simulink model "heli"  (R2020a)
settings: Solver=FixedStepAuto  StartTime=0  StopTime=Ts  FixedStep=0.0025  MaxStep=0.01  RelTol=1e-3  AbsTol=1e-3
values from neighbouring files (symbols this model uses):
  A_Fxyz_uvw_pqr = A([1 2 3],[1 2 3 4 5 6])    [heli_init.m]
  A_Mxyz_uvw_pqr = A([4 5 6],[1 2 3 4 5 6])    [heli_init.m]
  B_Fxyz_u_cont = B([1 2 3],[1 2 3 4])    [heli_init.m]
  B_Mxyz_u_cont = B([4 5 6],[1 2 3 4])    [heli_init.m]
  DCM_0 = [1 0 0 ... (first row only)    [heli_init.m]
  Dir_w = 0*[1 1 1 1 1 1]    [heli_init.m]
  East_0 = 0    [heli_init.m]
  h_0 = 0    [heli_init.m]
  hw = [0 200 5000 10000 15000 20000]    [heli_init.m]
  hw_gust = [0 1 h_island h_island+1 5000]    [heli_init.m]
  ic_euler_ang = zeros(3,1)    [heli_init.m]
  ic_U = sqrt(ic_u^2+ic_v^2+ic_w^2)    [heli_init.m]
  ic_v = 0.0000    (= 0)    [heli_init.m]
  ic_w = 0.0000    (= 0)    [heli_init.m]
  K_gust = 0    [heli_init.m]
  K_gust_factor = [1.1 1 .5 0.25 0]    [heli_init.m]
  M = 1    [heli_init.m]
  North_0 = 0    [heli_init.m]
  Pit_ic = 0    [heli_init.m]
  Psi = 353*pi/180.0    (= 6.16101225954)    [heli_init.m]
  Roll_ic = 0    [heli_init.m]
  Th_wind_limit = 40    [heli_init.m]
  Vw = 15*[1 1 1 1 1 1]    [heli_init.m]
  W_GUST = .8    (= 0.8)    [heli_init.m]
libraries: aerolibobsolete x2, AP_Conector x2, aerolibasang x1, aerolibwind2 x1

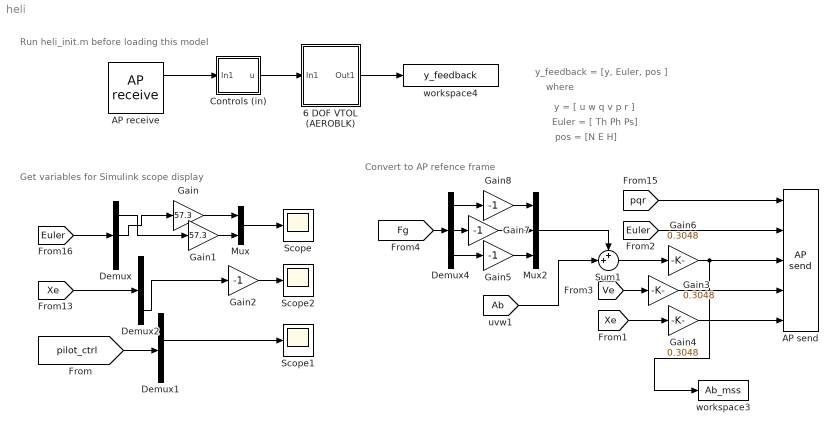
== system heli ==
  note: Run heli_init.m before loading this model
  note: Convert to AP refence frame
  note: Get variables for Simulink scope display
  note: y_feedback = [y, Euler, pos ]
  note: pos = [N E H]
  note: Euler = [ Th Ph Ps]
  note: y = [ u w q v p r ]
  note: where
  6 DOF VTOL (AEROBLK) : Subsystem
  AP receive : AP_Conector/AP receive  SystemSampleTime=-1  Latency=0  AutoFrameSizeCalculation=off
  AP send : AP_Conector/AP send  SystemSampleTime=-1  Latency=0  AutoFrameSizeCalculation=off
  Controls (in) : Subsystem
  Demux : Demux  Outputs=3
  Demux1 : Demux
  Demux2 : Demux  Outputs=3
  Demux4 : Demux  Outputs=3
  Gain : Gain  Gain=57.3
  Gain1 : Gain  Gain=57.3
  Gain{2,5,7..8} (4 alike) : Gain  Gain=-1
  Gain3 : Gain  Gain=0.3048
  Gain4 : Gain  Gain=0.3048
  Gain6 : Gain  Gain=0.3048
  Mux : Mux  Inputs=2
  Mux2 : Mux  Inputs=3
  Scope : Scope
  Scope1 : Scope
  Scope2 : Scope
  Sum1 : Sum  Inputs=++|
  workspace3 : ToWorkspace  VariableName=Ab_mss
  workspace4 : ToWorkspace  VariableName=y_feedback
  wires:
  Controls (in)/1(u) -> 6 DOF VTOL (AEROBLK)/1(In1)
  6 DOF VTOL (AEROBLK)/1(Out1) -> workspace4/1
  [Euler] -> Demux/1
  Demux/1 -> Gain1/1
  Demux/2 -> Gain/1
  Mux/1 -> Scope/1
  [pilot_ctrl] -> Demux1/1
  Demux1/2 -> Scope1/1
  [Xe] -> Demux2/1
  Demux2/3 -> Gain2/1
  Gain/1 -> Mux/1
  Gain1/1 -> Mux/2
  Gain2/1 -> Scope2/1
  [pqr] -> AP send/1
  [Euler] -> AP send/2
  [Ve] -> Gain3/1
  [Xe] -> Gain4/1
  Gain3/1 -> AP send/4
  Gain4/1 -> AP send/5
  [Ab] -> Sum1/2
  [Fg] -> Demux4/1
  Demux4/1 -> Gain8/1
  Demux4/2 -> Gain7/1
  Mux2/1 -> Sum1/1
  Gain5/1 -> Mux2/3
  Demux4/3 -> Gain5/1
  Sum1/1 -> Gain6/1
  Gain6/1 -> workspace3/1, AP send/3
  Gain8/1 -> Mux2/1
  Gain7/1 -> Mux2/2
  AP receive/1 -> Controls (in)/1(In1)

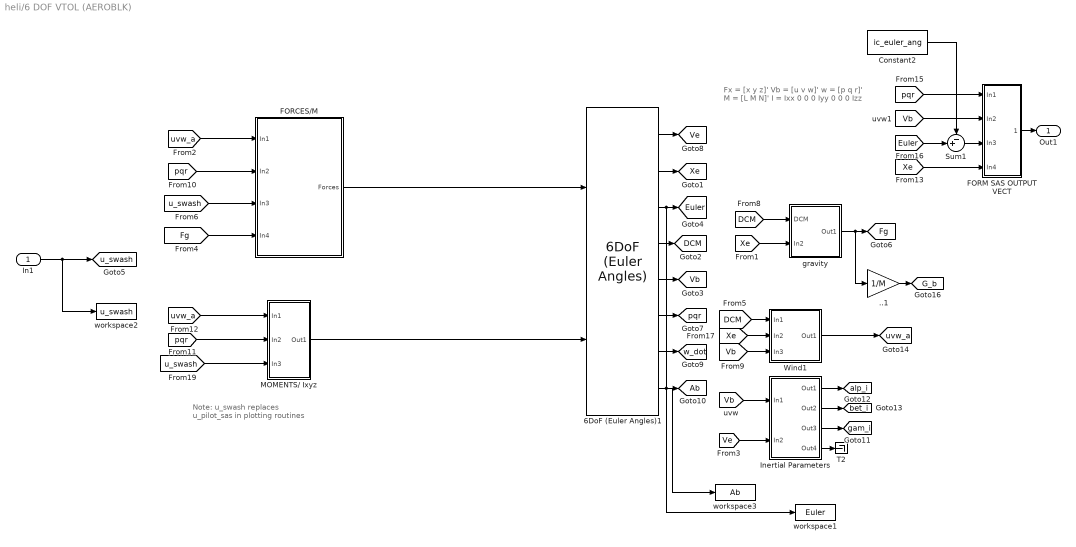
== system heli/6 DOF VTOL (AEROBLK) ==
  note: Fx = [x y z]'
      |
      | Vb = [u v w]'
      |
      | w = [p q r]'
      |
      | M = [L M N]'
      |
      | I =  Ixx  0     0
      |      0   Iyy    0
      |        	  0   0    Izz
  note: Note: u_swash replaces
      |  u_pilot_sas in plotting routines
  In1 : Inport
  ..1 : Gain  Gain=1/M  SaturateOnIntegerOverflow=on  OutDataTypeStr=Inherit: Same as input  ParamDataTypeStr=Inherit: Same as input
  6DoF (Euler Angles)1 : aerolibobsolete/6DoF (Euler Angles)  units=English (Velocity in ft/s)  mtype=Fixed  rep=Euler Angles  xme_0=[North_0 East_0 -h_0]  Vm_0="[ic_U  ic_v  ic_w]"  eul_0="[Roll_ic  Pit_ic  Psi]"  pm_0=[0 0 0]  mass_0=1  mass_e=0.5  mass_f=2.0  inertia=eye(3)  inertia_e=eye(3)  inertia_f=2*eye(3)  k_quat=1.0
      link override Calculate DCM & Euler Angles/phi theta psi: InitialCondition=[0,0,0]
  Constant2 : Constant  Value=ic_euler_ang
  FORCES/M : Subsystem
  FORM SAS OUTPUT VECT : Subsystem
  Inertial Parameters : Subsystem
  "MOMENTS/ Ixyz " : Subsystem
  Sum1 : Sum  Inputs=-+|
  T2 : Terminator
  Wind1 : Subsystem
  gravity : Subsystem
  workspace1 : ToWorkspace  VariableName=Euler
  workspace2 : ToWorkspace  VariableName=u_swash
  workspace3 : ToWorkspace  VariableName=Ab
  Out1 : Outport  VectorParamsAs1DForOutWhenUnconnected=off
  tag scope: Ab=global, DCM=global, Euler=global, Fg=global, G_b=global, Vb=global, Ve=global, Xe=global, alp_i=global, bet_i=global, gam_i=global, pqr=global, u_swash=global, uvw_a=global, w_dot=global
  wires:
  [pqr] -> "MOMENTS/ Ixyz "/2(In2)
  [uvw_a] -> "MOMENTS/ Ixyz "/1(In1)
  In1/1 -> workspace2/1, [u_swash]
  [Vb] -> Inertial Parameters/1(In1)
  [Ve] -> Inertial Parameters/2(In2)
  Inertial Parameters/3(Out3) -> [gam_i]
  Inertial Parameters/1(Out1) -> [alp_i]
  Inertial Parameters/2(Out2) -> [bet_i]
  Inertial Parameters/4(Out4) -> T2/1
  [Xe] -> Wind1/2(In2)
  [DCM] -> Wind1/1(In1)
  [Vb] -> Wind1/3(In3)
  [pqr] -> FORM SAS OUTPUT VECT/1(In1)
  [Vb] -> FORM SAS OUTPUT VECT/2(In2)
  [Xe] -> FORM SAS OUTPUT VECT/4(In4)
  FORM SAS OUTPUT VECT/1(Out1) -> Out1/1
  6DoF (Euler Angles)1/1 -> [Ve]
  6DoF (Euler Angles)1/2 -> [Xe]
  6DoF (Euler Angles)1/4 -> [DCM]
  6DoF (Euler Angles)1/5 -> [Vb]
  6DoF (Euler Angles)1/6 -> [pqr]
  6DoF (Euler Angles)1/7 -> [w_dot]
  6DoF (Euler Angles)1/8 -> workspace3/1, [Ab]
  Sum1/1 -> FORM SAS OUTPUT VECT/3(In3)
  [pqr] -> FORCES/M/2(In2)
  [u_swash] -> FORCES/M/3(In3)
  gravity/1(Out1) -> ..1/1, [Fg]
  [Xe] -> gravity/2(In2)
  [DCM] -> gravity/1(DCM)
  ..1/1 -> [G_b]
  [u_swash] -> "MOMENTS/ Ixyz "/3(In3)
  6DoF (Euler Angles)1/3 -> workspace1/1, [Euler]
  FORCES/M/1(Forces) -> 6DoF (Euler Angles)1/1
  [uvw_a] -> FORCES/M/1(In1)
  "MOMENTS/ Ixyz "/1(Out1) -> 6DoF (Euler Angles)1/2
  Wind1/1(Out1) -> [uvw_a]
  [Fg] -> FORCES/M/4(In4)
  Constant2/1 -> Sum1/1
  [Euler] -> Sum1/2

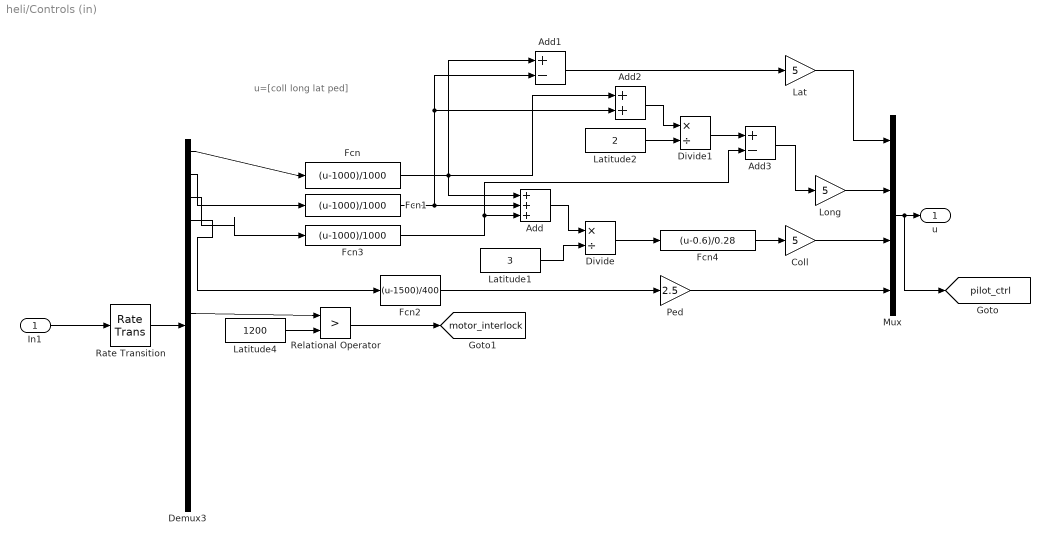
== system heli/Controls (in) ==
  note: u=[coll long lat ped]
  In1 : Inport
  Add : Sum  Inputs=+++
  Add1 : Sum  Inputs=+-
  Add2 : Sum
  Add3 : Sum  Inputs=+-
  Coll : Gain  Gain=5
  Demux3 : Demux  Outputs=16
  Divide : Product  Inputs=*/
  Divide1 : Product  Inputs=*/
  Fcn : Fcn  Expr=(u-1000)/1000
  Fcn1 : Fcn  Expr=(u-1000)/1000
  Fcn2 : Fcn  Expr=(u-1500)/400
  Fcn3 : Fcn  Expr=(u-1000)/1000
  Fcn4 : Fcn  Expr=(u-0.6)/0.28
  Lat : Gain  Gain=5
  Latitude1 : Constant  Value=3
  Latitude2 : Constant  Value=2
  Latitude4 : Constant  Value=1200
  Long : Gain  Gain=5
  Mux : Mux
  Ped : Gain  Gain=2.5
  Rate Transition : RateTransition
  Relational Operator : RelationalOperator  Operator=>  OutDataTypeStr=boolean  RndMeth=Simplest
  u : Outport  VectorParamsAs1DForOutWhenUnconnected=off
  tag scope: motor_interlock=global, pilot_ctrl=global
  wires:
  Fcn2/1 -> Ped/1
  Mux/1 -> [pilot_ctrl], u/1
  Coll/1 -> Mux/3
  Lat/1 -> Mux/1
  Long/1 -> Mux/2
  Ped/1 -> Mux/4
  Demux3/3 -> Fcn3/1
  Demux3/4 -> Fcn2/1
  Demux3/1 -> Fcn/1
  Demux3/2 -> Fcn1/1
  Rate Transition/1 -> Demux3/1
  In1/1 -> Rate Transition/1
  Demux3/8 -> Relational Operator/1
  Latitude4/1 -> Relational Operator/2
  Relational Operator/1 -> [motor_interlock]
  Fcn/1 -> Add/1, Add1/1, Add2/1
  Fcn1/1 -> Add2/2, Add1/2, Add/2
  Fcn3/1 -> Add3/2, Add/3
  Add/1 -> Divide/1
  Latitude1/1 -> Divide/2
  Divide/1 -> Fcn4/1
  Fcn4/1 -> Coll/1
  Add1/1 -> Lat/1
  Add2/1 -> Divide1/1
  Latitude2/1 -> Divide1/2
  Divide1/1 -> Add3/1
  Add3/1 -> Long/1

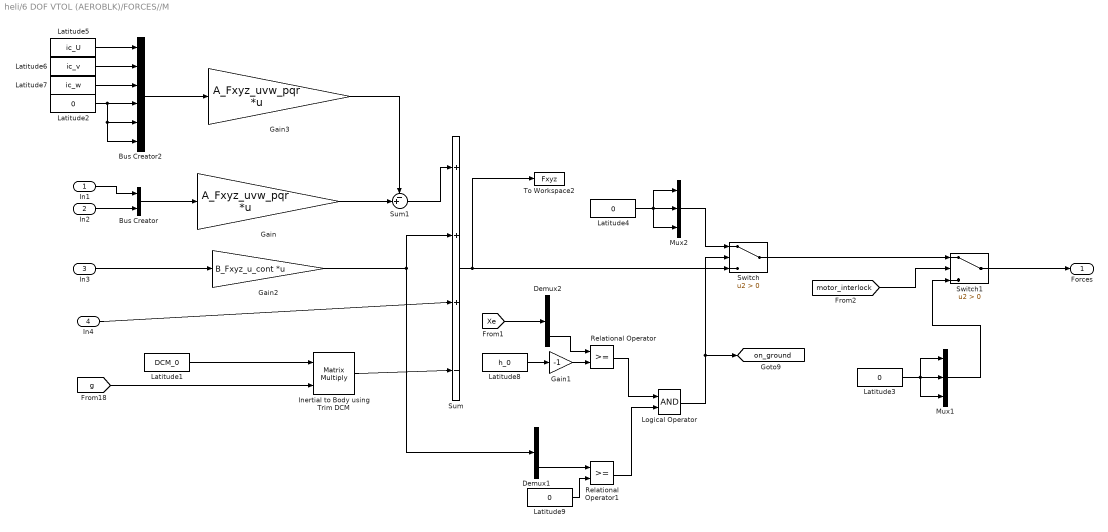
== system heli/6 DOF VTOL (AEROBLK)/FORCES//M ==
  In1 : Inport
  In2 : Inport  Port=2
  In3 : Inport  Port=3
  In4 : Inport  Port=4
  Bus Creator : BusCreator  Inputs=2
  Bus Creator2 : BusCreator  Inputs=6
  Demux1 : Demux  Outputs=3
  Demux2 : Demux  Outputs=3
  Gain : Gain  Gain=A_Fxyz_uvw_pqr  Multiplication=Matrix(K*u) (u vector)
  Gain1 : Gain  Gain=-1
  Gain2 : Gain  Gain=B_Fxyz_u_cont  Multiplication=Matrix(K*u) (u vector)
  Gain3 : Gain  Gain=A_Fxyz_uvw_pqr  Multiplication=Matrix(K*u) (u vector)
  Inertial to Body using Trim DCM : Product  Multiplication=Matrix(*)  InputSameDT=on  SaturateOnIntegerOverflow=on  OutDataTypeStr=Inherit: Same as first input
  Latitude1 : Constant  Value=DCM_0
  Latitude{2..4,9} (4 alike) : Constant  Value=0
  Latitude5 : Constant  Value=ic_U
  Latitude6 : Constant  Value=ic_v
  Latitude7 : Constant  Value=ic_w
  Latitude8 : Constant  Value=h_0
  Logical Operator : Logic  AllPortsSameDT=off  OutDataTypeStr=boolean
  Mux1 : Mux  Inputs=3
  Mux2 : Mux  Inputs=3
  Relational Operator : RelationalOperator  OutDataTypeStr=boolean  RndMeth=Simplest
  Relational Operator1 : RelationalOperator  OutDataTypeStr=boolean  RndMeth=Simplest
  Sum : Sum  Inputs=|+++-
  Sum1 : Sum  Inputs=-+|
  Switch : Switch  Criteria=u2 > Threshold
  Switch1 : Switch  Criteria=u2 > Threshold
  To Workspace2 : ToWorkspace  VariableName=Fxyz  SampleTime=-1
  Forces : Outport  VectorParamsAs1DForOutWhenUnconnected=off
  tag scope: on_ground=global
  wires:
  In3/1 -> Gain2/1
  In2/1 -> Bus Creator/2
  Sum/1 -> Switch/3, To Workspace2/1
  Gain2/1 -> Demux1/1, Sum/2
  Bus Creator/1 -> Gain/1
  Sum1/1 -> Sum/1
  Bus Creator2/1 -> Gain3/1
  Latitude5/1 -> Bus Creator2/1
  Latitude6/1 -> Bus Creator2/2
  Latitude7/1 -> Bus Creator2/3
  Latitude2/1 -> Bus Creator2/4, Bus Creator2/5, Bus Creator2/6
  Gain3/1 -> Sum1/1
  Gain/1 -> Sum1/2
  In1/1 -> Bus Creator/1
  [g] -> Inertial to Body using Trim DCM/2
  In4/1 -> Sum/3
  Latitude1/1 -> Inertial to Body using Trim DCM/1
  Inertial to Body using Trim DCM/1 -> Sum/4
  Switch/1 -> Switch1/1
  [Xe] -> Demux2/1
  Demux2/3 -> Relational Operator/1
  Latitude8/1 -> Gain1/1
  Demux1/3 -> Relational Operator1/1
  Latitude9/1 -> Relational Operator1/2
  Relational Operator/1 -> Logical Operator/1
  Relational Operator1/1 -> Logical Operator/2
  Latitude4/1 -> Mux2/1, Mux2/3, Mux2/2
  Mux2/1 -> Switch/1
  Gain1/1 -> Relational Operator/2
  [motor_interlock] -> Switch1/2
  Logical Operator/1 -> [on_ground], Switch/2
  Mux1/1 -> Switch1/3
  Latitude3/1 -> Mux1/1, Mux1/3, Mux1/2
  Switch1/1 -> Forces/1

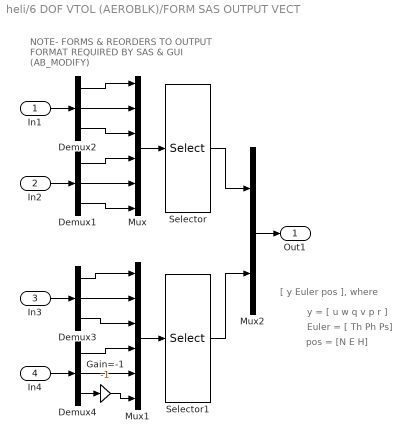
== system heli/6 DOF VTOL (AEROBLK)/FORM SAS OUTPUT VECT ==
  note: NOTE- FORMS & REORDERS TO OUTPUT FORMAT
      | REQUIRED BY SAS & GUI (AB_MODIFY)
  note: [ y Euler pos ], where
  note: pos = [N E H]
  note: Euler = [ Th Ph Ps]
  note: y = [ u w q v p r ]
  In1 : Inport
  In2 : Inport  Port=2
  In3 : Inport  Port=3
  In4 : Inport  Port=4
  Demux{1..4} (4 alike) : Demux  Outputs=3
  Gain=-1 : Gain  Gain=-1
  Mux : Mux  Inputs=6
  Mux1 : Mux  Inputs=6
  Mux2 : Mux  Inputs=2
  Selector : Selector  InputPortWidth=6  IndexOptions=Index vector (dialog)  Indices=[4 6 2 5 1 3]  OutputSizes=1
  Selector1 : Selector  InputPortWidth=6  IndexOptions=Index vector (dialog)  Indices=[2 1 3 4 5 6]  OutputSizes=1
  Out1 : Outport  VectorParamsAs1DForOutWhenUnconnected=off
  wires:
  Demux2/1 -> Mux/1
  Demux2/2 -> Mux/2
  Demux1/1 -> Mux/4
  Demux1/2 -> Mux/5
  Demux1/3 -> Mux/6
  Mux/1 -> Selector/1
  Demux2/3 -> Mux/3
  Mux1/1 -> Selector1/1
  Selector/1 -> Mux2/1
  Selector1/1 -> Mux2/2
  Demux3/1 -> Mux1/1
  Demux3/2 -> Mux1/2
  Demux3/3 -> Mux1/3
  Demux4/1 -> Mux1/4
  Demux4/2 -> Mux1/5
  Gain=-1/1 -> Mux1/6
  Demux4/3 -> Gain=-1/1
  In1/1 -> Demux2/1
  In2/1 -> Demux1/1
  Mux2/1 -> Out1/1
  In3/1 -> Demux3/1
  In4/1 -> Demux4/1

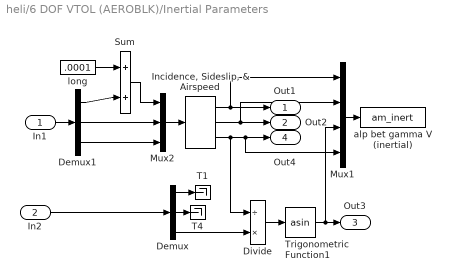
== system heli/6 DOF VTOL (AEROBLK)/Inertial Parameters ==
  In1 : Inport
  In2 : Inport  Port=2
  Demux : Demux  Outputs=3
  Demux1 : Demux  Outputs=3
  Divide : Product  Inputs=/*
  "Incidence, Sideslip, & Airspeed" : aerolibasang/Incidence, Sideslip, & Airspeed
  Mux1 : Mux
  Mux2 : Mux  Inputs=3
  Sum : Sum  Inputs=|++
  T1 : Terminator
  T4 : Terminator
  Trigonometric Function1 : Trigonometry  Operator=asin
  alp bet gamma V (inertial) : ToWorkspace  VariableName=am_inert  SampleTime=-1
  long : Constant  Value=.0001
  Out1 : Outport  VectorParamsAs1DForOutWhenUnconnected=off
  Out2 : Outport  Port=2  VectorParamsAs1DForOutWhenUnconnected=off
  Out3 : Outport  Port=3  VectorParamsAs1DForOutWhenUnconnected=off
  Out4 : Outport  Port=4  VectorParamsAs1DForOutWhenUnconnected=off
  wires:
  Divide/1 -> Trigonometric Function1/1
  Demux/1 -> T1/1
  Demux/2 -> T4/1
  "Incidence, Sideslip, & Airspeed"/3 -> Divide/1, Out4/1, Mux1/4
  Demux/3 -> Divide/2
  "Incidence, Sideslip, & Airspeed"/1 -> Out1/1, Mux1/1
  "Incidence, Sideslip, & Airspeed"/2 -> Out2/1, Mux1/2
  Trigonometric Function1/1 -> Out3/1, Mux1/3
  In1/1 -> Demux1/1
  Mux2/1 -> "Incidence, Sideslip, & Airspeed"/1
  Demux1/2 -> Mux2/2
  Demux1/3 -> Mux2/3
  In2/1 -> Demux/1
  long/1 -> Sum/1
  Demux1/1 -> Sum/2
  Sum/1 -> Mux2/1
  Mux1/1 -> alp bet gamma V (inertial)/1

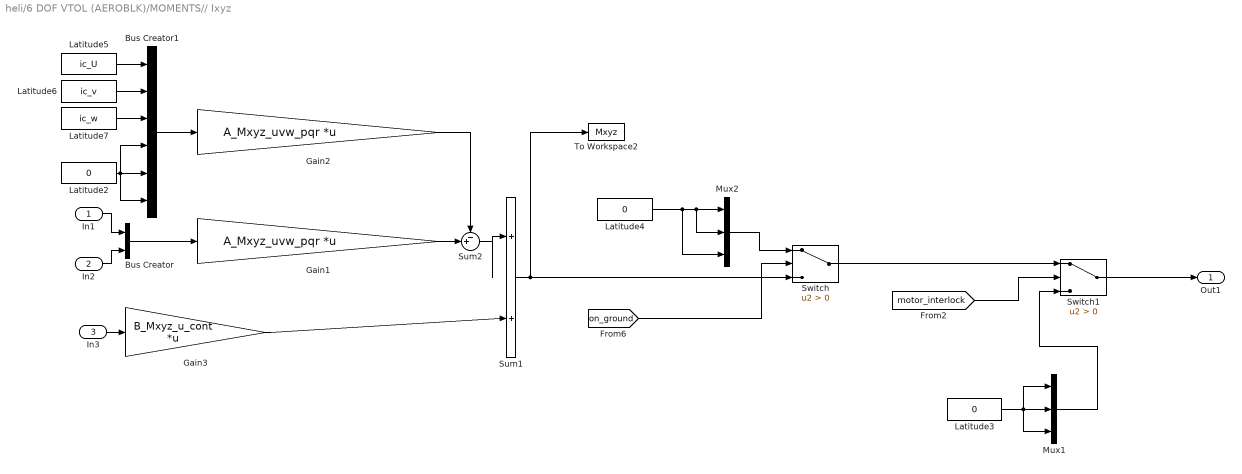
== system heli/6 DOF VTOL (AEROBLK)/MOMENTS// Ixyz  ==
  In1 : Inport
  In2 : Inport  Port=2
  In3 : Inport  Port=3
  Bus Creator : BusCreator  Inputs=2
  Bus Creator1 : BusCreator  Inputs=6
  Gain1 : Gain  Gain=A_Mxyz_uvw_pqr  Multiplication=Matrix(K*u) (u vector)
  Gain2 : Gain  Gain=A_Mxyz_uvw_pqr  Multiplication=Matrix(K*u) (u vector)
  Gain3 : Gain  Gain=B_Mxyz_u_cont  Multiplication=Matrix(K*u) (u vector)
  Latitude2 : Constant  Value=0
  Latitude3 : Constant  Value=0
  Latitude4 : Constant  Value=0
  Latitude5 : Constant  Value=ic_U
  Latitude6 : Constant  Value=ic_v
  Latitude7 : Constant  Value=ic_w
  Mux1 : Mux  Inputs=3
  Mux2 : Mux  Inputs=3
  Sum1 : Sum  Inputs=|++
  Sum2 : Sum  Inputs=-+|
  Switch : Switch  Criteria=u2 > Threshold
  Switch1 : Switch  Criteria=u2 > Threshold
  To Workspace2 : ToWorkspace  VariableName=Mxyz  SampleTime=-1
  Out1 : Outport  VectorParamsAs1DForOutWhenUnconnected=off
  wires:
  Sum1/1 -> Switch/3, To Workspace2/1
  In3/1 -> Gain3/1
  Bus Creator/1 -> Gain1/1
  Bus Creator1/1 -> Gain2/1
  Latitude2/1 -> Bus Creator1/5, Bus Creator1/4, Bus Creator1/6
  Latitude7/1 -> Bus Creator1/3
  Latitude6/1 -> Bus Creator1/2
  Latitude5/1 -> Bus Creator1/1
  Gain1/1 -> Sum2/2
  Gain2/1 -> Sum2/1
  Sum2/1 -> Sum1/1
  Gain3/1 -> Sum1/2
  In2/1 -> Bus Creator/2
  In1/1 -> Bus Creator/1
  [on_ground] -> Switch/2
  Mux2/1 -> Switch/1
  Latitude4/1 -> Mux2/3, Mux2/2, Mux2/1
  Switch/1 -> Switch1/1
  Switch1/1 -> Out1/1
  Latitude3/1 -> Mux1/1, Mux1/3, Mux1/2
  [motor_interlock] -> Switch1/2
  Mux1/1 -> Switch1/3

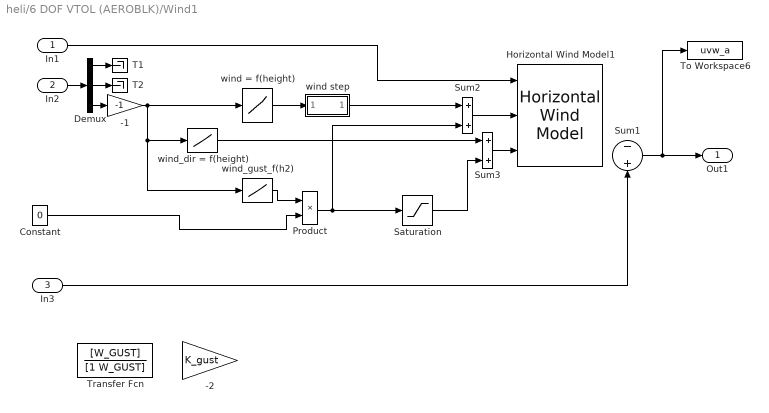
== system heli/6 DOF VTOL (AEROBLK)/Wind1 ==
  In1 : Inport
  In2 : Inport  Port=2
  In3 : Inport  Port=3
  -1 : Gain  Gain=-1
  -2 : Gain  Gain=K_gust
  Constant : Constant  Value=0
  Demux : Demux  Outputs=3
  Horizontal Wind Model1 : aerolibwind2/Horizontal Wind Model  units=English (Velocity in ft/s)  Vw_source=External  Vwind=0  W_source=External  Wdeg=0
  Product : Product  RndMeth=Zero
  Saturation : Saturate  UpperLimit=Th_wind_limit  LowerLimit=-Th_wind_limit
  Sum1 : Sum  Inputs=-+
  Sum2 : Sum
  Sum3 : Sum
  T1 : Terminator
  T2 : Terminator
  To Workspace6 : ToWorkspace  VariableName=uvw_a  SampleTime=-1
  Transfer Fcn : TransferFcn  Numerator=[W_GUST]  Denominator=[1 W_GUST]
  wind = f(height) : Lookup  InputValues=hw  Table=Vw
  wind step : Subsystem
  wind_dir = f(height) : Lookup  InputValues=hw  Table=Dir_w
  wind_gust_f(h2) : Lookup  InputValues=hw_gust  Table=K_gust_factor  LookUpMeth=Use Input Nearest
  Out1 : Outport  VectorParamsAs1DForOutWhenUnconnected=off
  wires:
  Demux/1 -> T1/1
  Demux/2 -> T2/1
  In1/1 -> Horizontal Wind Model1/1
  In2/1 -> Demux/1
  Sum1/1 -> To Workspace6/1, Out1/1
  -1/1 -> wind_dir = f(height)/1, wind_gust_f(h2)/1, wind = f(height)/1
  Demux/3 -> -1/1
  Sum2/1 -> Horizontal Wind Model1/2
  ? -> ?
  Saturation/1 -> Sum3/2
  wind_dir = f(height)/1 -> Sum3/1
  Sum3/1 -> Horizontal Wind Model1/3
  Constant/1 -> Product/2
  wind_gust_f(h2)/1 -> Product/1
  Product/1 -> Saturation/1, Sum2/2
  wind = f(height)/1 -> wind step/1(In1)
  wind step/1(Out1) -> Sum2/1
  In3/1 -> Sum1/2

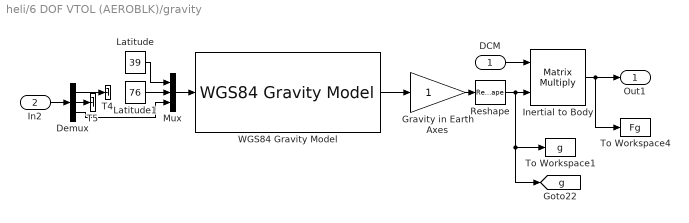
== system heli/6 DOF VTOL (AEROBLK)/gravity ==
  DCM : Inport
  In2 : Inport  Port=2
  Demux : Demux  Outputs=3
  Gravity in Earth Axes : Gain  SaturateOnIntegerOverflow=on  OutDataTypeStr=Inherit: Same as input  ParamDataTypeStr=Inherit: Same as input
  Inertial to Body : Product  Multiplication=Matrix(*)  InputSameDT=on  SaturateOnIntegerOverflow=on  OutDataTypeStr=Inherit: Same as first input
  Latitude : Constant  Value=39
  Latitude1 : Constant  Value=76
  Mux : Mux  Inputs=3
  Reshape : Reshape
  T4 : Terminator
  T5 : Terminator
  To Workspace1 : ToWorkspace  VariableName=g  SampleTime=-1
  To Workspace4 : ToWorkspace  VariableName=Fg  SampleTime=-1
  "WGS84 Gravity Model " : aerolibobsolete/WGS84 Gravity Model   model=WGS84 Exact  units=English  no_atmos=on  precessing=on  jd_loc=off  month=October  day=10  year=2004  no_centrifugal=on  action=None
  Out1 : Outport  VectorParamsAs1DForOutWhenUnconnected=off
  tag scope: g=global
  wires:
  In2/1 -> Demux/1
  Demux/2 -> T5/1
  Demux/1 -> T4/1
  Inertial to Body/1 -> To Workspace4/1, Out1/1
  DCM/1 -> Inertial to Body/1
  Gravity in Earth Axes/1 -> Reshape/1
  "WGS84 Gravity Model "/1 -> Gravity in Earth Axes/1
  Mux/1 -> "WGS84 Gravity Model "/1
  Reshape/1 -> Inertial to Body/2, To Workspace1/1, [g]
  Latitude1/1 -> Mux/2
  Latitude/1 -> Mux/1
  Demux/3 -> Mux/3

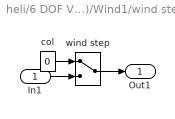
== system heli/6 DOF VTOL (AEROBLK)/Wind1/wind step ==
  In1 : Inport
  col : Constant  Value=0
  wind step : ManualSwitch
  Out1 : Outport  VectorParamsAs1DForOutWhenUnconnected=off
  wires:
  col/1 -> wind step/1
  wind step/1 -> Out1/1
  In1/1 -> wind step/2
